simulink model "AcceleratorOld"  (R2019a)
settings: Solver=FixedStepAuto  StartTime=0.0  StopTime=20  FixedStep=step  RelTol=1e-3
model workspace (MAT data in the model file):
  a = Simulink.Signal
  a.DataType = 'double'
  a.DocUnits = 'rad/S^2'
  a.Dimensions = 1
  a.DimensionsMode = 'Fixed'
  a.Complexity = 'real'
  a.SampleTime = -1
  a.SamplingMode = 'auto'
  a.InitialValue = '0'
  d = Simulink.Signal
  d.DataType = 'double'
  d.DocUnits = 'rad'
  d.Dimensions = 1
  d.DimensionsMode = 'Fixed'
  d.Complexity = 'real'
  d.SampleTime = -1
  d.SamplingMode = 'auto'
  d.InitialValue = '0'
  j = Simulink.Signal
  j.DataType = 'double'
  j.DocUnits = 'rad/S^3'
  j.Dimensions = 1
  j.DimensionsMode = 'Fixed'
  j.Complexity = 'real'
  j.SampleTime = -1
  j.SamplingMode = 'auto'
  j.InitialValue = '1000'
  step = 0.001
  t_AASearch = Simulink.Signal
  t_AASearch.Description = 'This variable is the searching tolernece for DS.'
  t_AASearch.DataType = 'double'
  t_AASearch.DocUnits = 'm'
  t_AASearch.Dimensions = 1
  t_AASearch.DimensionsMode = 'auto'
  t_AASearch.Complexity = 'real'
  t_AASearch.SampleTime = -1
  t_AASearch.SamplingMode = 'auto'
  t_AASearch.InitialValue = '0.001'
  v = Simulink.Signal
  v.DataType = 'double'
  v.Dimensions = 1
  v.DimensionsMode = 'auto'
  v.Complexity = 'real'
  v.SampleTime = -1
  v.SamplingMode = 'auto'
  v.InitialValue = '0'
settings Model: OrderedModelArguments=off  Creator=EiLit  LastModifiedBy=EiLit
settings DataIOCC: ReturnWorkspaceOutputs=off
settings DebuggingCC: ReadBeforeWriteMsg=EnableAllAsWarning  WriteAfterWriteMsg=EnableAllAsWarning  WriteAfterReadMsg=EnableAllAsWarning  ArithmeticOperatorsInVariantConditions=warning

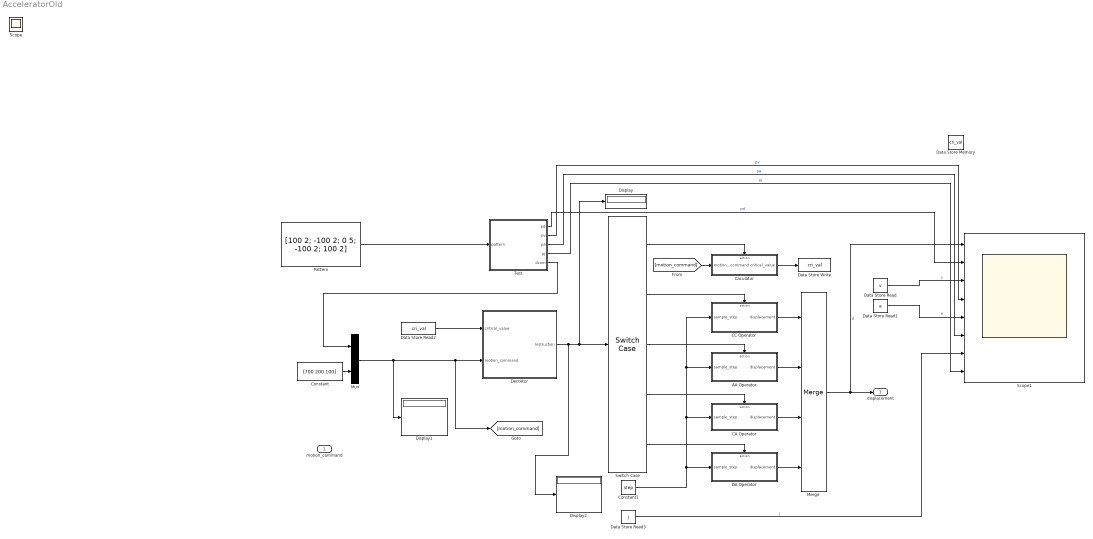
== system AcceleratorOld ==
  motion_command : Inport
  AA Operator : Subsystem  TreatAsAtomicUnit=on
  CA Operator : Subsystem  TreatAsAtomicUnit=on
  CC Operator : Subsystem  TreatAsAtomicUnit=on
  Caculator : Subsystem  TreatAsAtomicUnit=on
  Constant : Constant  Value=[700 200 100]
  Constant1 : Constant  Value=step
  DA Operator : Subsystem  TreatAsAtomicUnit=on
  Data Store Memory : DataStoreMemory  DataStoreName=cri_val  ReadBeforeWriteMsg=warning  WriteAfterWriteMsg=warning  WriteAfterReadMsg=warning  InitialValue=zeros(8,4)  ShowAdditionalParam=off
  Data Store Read : DataStoreRead  DataStoreName=v
  Data Store Read1 : DataStoreRead  DataStoreName=a
  Data Store Read2 : DataStoreRead  DataStoreName=cri_val
  Data Store Read3 : DataStoreRead  DataStoreName=j
  Data Store Write : DataStoreWrite  DataStoreName=cri_val
  Dectetor : Subsystem
  Display : Display
  Display1 : Display
  Display2 : Display
  Merge : Merge  Inputs=4  InitialOutput=[0]
  Mux : Mux  Inputs=2
  Pattern : Constant  Value=[100 2; -100 2; 0 5; -100 2; 100 2]  VectorParams1D=off
  Scope1 : Scope  NumInputPorts=8
  Switch Case : SwitchCase  CaseConditions={0,1,2,3,4}  ShowDefaultCase=off
  Test : Subsystem
  displacement : Outport
  Scope : Scope
  wires:
  Test/5(dcom) -> Mux/1
  AA Operator/1(displacement) -> Merge/2
  CC Operator/1(displacement) -> Merge/1
  Switch Case/1 -> Caculator/Action
  Data Store Read/1 -> Scope1/3  "v"
  Test/1(pd) -> Scope1/2  "pd"
  Data Store Read1/1 -> Scope1/5  "a"
  Dectetor/1(Instruction) -> Display2/1, Switch Case/1, Display/1
  Constant1/1 -> CC Operator/1(sample_step), AA Operator/1(sample_step), CA Operator/1(sample_step), DA Operator/1(sample_step)
  CA Operator/1(displacement) -> Merge/3
  DA Operator/1(displacement) -> Merge/4
  Data Store Read2/1 -> Dectetor/1(critical_value)
  Test/2(pv) -> Scope1/4  "pv"
  Switch Case/5 -> DA Operator/Action
  Merge/1 -> Scope1/1, displacement/1  "d"
  Switch Case/2 -> CC Operator/Action
  [motion_command] -> Caculator/1(motion_command)
  Caculator/1(critical_value) -> Data Store Write/1
  Constant/1 -> Mux/2
  Switch Case/3 -> AA Operator/Action
  Test/3(pa) -> Scope1/6  "pa"
  Mux/1 -> Display1/1, [motion_command], Dectetor/2(motion_command)
  Switch Case/4 -> CA Operator/Action
  Pattern/1 -> Test/1(pattern)
  Test/4(pj) -> Scope1/8  "pj"
  Data Store Read3/1 -> Scope1/7  "j"

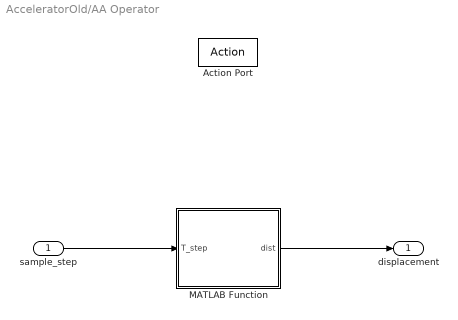
== system AcceleratorOld/AA Operator ==
  sample_step : Inport
  Action Port : ActionPort  ActionPortLabel=case [ 2 ]:
  MATLAB Function : MATLAB Function  TreatAsAtomicUnit=on
  displacement : Outport  PortDimensions=1
  wires:
  sample_step/1 -> MATLAB Function/1(T_step)
  MATLAB Function/1(dist) -> displacement/1

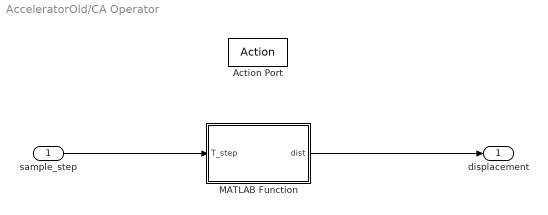
== system AcceleratorOld/CA Operator ==
  sample_step : Inport
  Action Port : ActionPort  ActionPortLabel=case [ 3 ]:
  MATLAB Function : MATLAB Function  TreatAsAtomicUnit=on
  displacement : Outport
  wires:
  sample_step/1 -> MATLAB Function/1(T_step)
  MATLAB Function/1(dist) -> displacement/1

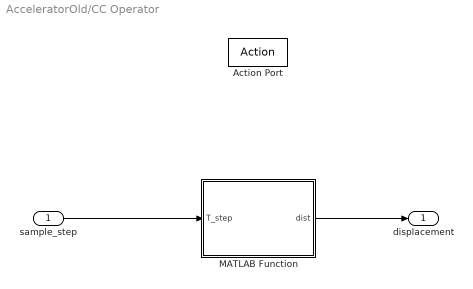
== system AcceleratorOld/CC Operator ==
  sample_step : Inport
  Action Port : ActionPort  ActionPortLabel=case [ 1 ]:
  MATLAB Function : MATLAB Function  TreatAsAtomicUnit=on
  displacement : Outport
  wires:
  MATLAB Function/1(dist) -> displacement/1
  sample_step/1 -> MATLAB Function/1(T_step)

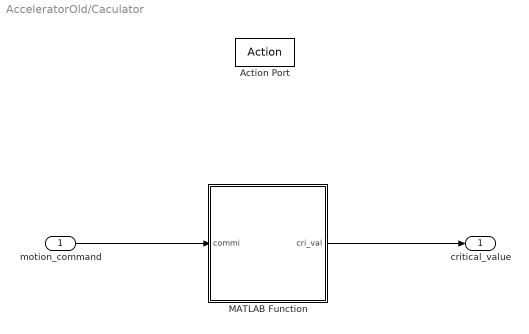
== system AcceleratorOld/Caculator ==
  motion_command : Inport
  Action Port : ActionPort  ActionPortLabel=case [ 0 ]:
  MATLAB Function : MATLAB Function  TreatAsAtomicUnit=on
  critical_value : Outport
  wires:
  motion_command/1 -> MATLAB Function/1(commi)
  MATLAB Function/1(cri_val) -> critical_value/1

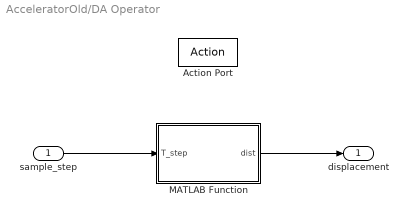
== system AcceleratorOld/DA Operator ==
  sample_step : Inport
  Action Port : ActionPort  ActionPortLabel=case [ 4 ]:
  MATLAB Function : MATLAB Function  TreatAsAtomicUnit=on
  displacement : Outport
  wires:
  sample_step/1 -> MATLAB Function/1(T_step)
  MATLAB Function/1(dist) -> displacement/1

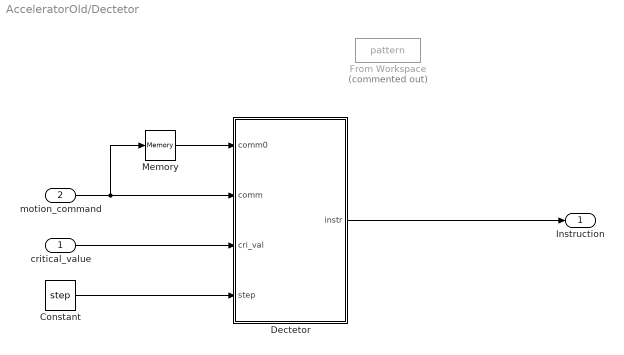
== system AcceleratorOld/Dectetor ==
  critical_value : Inport
  motion_command : Inport  Port=2
  Constant : Constant  Value=step
  Dectetor : MATLAB Function  TreatAsAtomicUnit=on
  From Workspace : FromWorkspace  Commented=on  VariableName=pattern  SampleTime=0
  Memory : Memory  InitialCondition=[0 0 0 0]
  Instruction : Outport
  wires:
  motion_command/1 -> Memory/1, Dectetor/2(comm)
  Dectetor/1(instr) -> Instruction/1
  critical_value/1 -> Dectetor/3(cri_val)
  Memory/1 -> Dectetor/1(comm0)
  Constant/1 -> Dectetor/4(step)

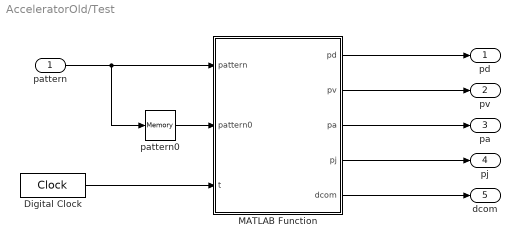
== system AcceleratorOld/Test ==
  pattern : Inport
  Digital Clock : DigitalClock  SampleTime=0.001
  MATLAB Function : MATLAB Function  TreatAsAtomicUnit=on
  pattern0 : Memory
  pd : Outport
  pv : Outport  Port=2
  pa : Outport  Port=3
  pj : Outport  Port=4
  dcom : Outport  Port=5
  wires:
  pattern/1 -> MATLAB Function/1(pattern), pattern0/1
  MATLAB Function/1(pd) -> pd/1
  pattern0/1 -> MATLAB Function/2(pattern0)
  Digital Clock/1 -> MATLAB Function/3(t)
  MATLAB Function/4(pj) -> pj/1
  MATLAB Function/3(pa) -> pa/1
  MATLAB Function/2(pv) -> pv/1
  MATLAB Function/5(dcom) -> dcom/1

== matlab function AcceleratorOld/Dectetor/Dectetor ==
  data: comm0 input; comm input; instr output; cri_val input; d data_store_memory; v data_store_memory; a data_store_memory; step input; j data_store_memory
function instr = fcn(comm0, comm, cri_val, step)
%% Initialization
global d v a j
persistent phasei

instr = 0;

if isempty(phasei)
    phasei = 0;
end

% i stands for ith step:
% step 0: pre-Acc step;
% step 1: 1st Acc step;
% step 2: 1st CA step;
% step 3: 1st Dec step;
% ...

% Judge the direction
dir = comm(1)/abs(comm(1));
comm(2:4) = dir * comm(2:4);
commabs = abs(comm);            % Absolute command value used to calculate the neighbor.

%% Determine the instruction
if ~(comm == comm0)                % If need to re-calculate the critical value.
    instr = 0;
    j = 0;
    phasei = 0;
else
    temp1 = cri_val(2,3) - commabs(4) * step;      % The neighbor of the critical value used to take care of the direction of acceleration of the 1st step
    temp2 = cri_val(2,3) + commabs(4) * step;
    switch phasei
        case 0
            if cri_val(1,3)==0    % If there is pre-Acc step exist (or intially 0)
                if a*(a+comm(4)*step) >= 0    %If the pre-Acc step finished
                    [d, v, a, j, phasei, instr] = instrGen(step, dir, phasei, instr, cri_val, comm, commabs, temp1, temp2);
                else                        %If the pre-Acc step not finished
                    instr = 2;
                    j = -comm(4);
                end
            else                            %If the pre-Acc step does not exist
                [d, v, a, j, phasei, instr] = instrGen(step, dir, phasei, instr, cri_val, comm, commabs, temp1, temp2);
            end
        case 1
            if temp1<=a && a<=temp2                  % If a is in the neighbor, then step 1 is finished.
                [d, v, a, j, phasei, instr] = instrGen(step, dir, phasei, instr, cri_val, comm, commabs, temp1, temp2);
            else
                instr = 2;
                if a > cri_val(2,3)
                    j = -commabs(4);
                else
                    j = commabs(4);
                end
            end
        case 2
            temp = v + 0.5*comm(4)*step^2 + cri_val(3,3)*step;
            if dir * temp >= dir * cri_val(3,2)     % If velocity reaches the critical value
                [d, v, a, j, phasei, instr] = instrGen(step, dir, phasei, instr, cri_val, comm, commabs, temp1, temp2);
            else                                    % If velocity does not reach the critical value
                j = 0;
                instr = 3;
            end
        case 3
            temp = a - comm(4) * step;
            if dir * temp <= 0            % If acceleration is reduced to 0;
                [d, v, a, j, phasei, instr] = instrGen(step, dir, phasei, instr, cri_val, comm, commabs, temp1, temp2);
            else                                    % If acceleration is not reduced to 0;
                j = comm(4);
                instr = 4;
            end
        case 4
            temp = d + cri_val(5,2)*step;
            if dir * temp >= dir * cri_val(5,1)
                [d, v, a, j, phasei, instr] = instrGen(step, dir, phasei, instr, cri_val, comm, commabs, temp1, temp2);
            else
                j = 0;
                instr = 1;
            end
        case 5
            temp = a - comm(4) * step;
            if dir * temp <= dir * cri_val(6,3)
                [d, v, a, j, phasei, instr] = instrGen(step, dir, phasei, instr, cri_val, comm, commabs, temp1, temp2);
            else
                j = -comm(4);
                instr = 2;
            end
        case 6
            temp = v - 0.5*comm(4)*step^2 + cri_val(7,3)*step;
            if dir * temp <= cri_val(7,2)
                [d, v, a, j, phasei, instr] = instrGen(step, dir, phasei, instr, cri_val, comm, commabs, temp1, temp2);
            else
                j = 0;
                instr = 3;
            end
        case 7
            temp = a + comm(4) * step;
            if dir * temp >= 0
                [d, v, a, j, phasei, instr] = instrGen(step, dir, phasei, instr, cri_val, comm, commabs, temp1, temp2);
            else
                j = -comm(4);
                instr = 4;
            end
        otherwise
            instr = 1;
            j = 0;
    end
end
  
end

== matlab function AcceleratorOld/CC Operator/MATLAB Function ==
  data: T_step input; dist output; v data_store_memory; d data_store_memory; a data_store_memory
function dist = fcn(T_step)
global d v a
a = 0;
d = d + v*T_step;
dist = d;

== matlab function AcceleratorOld/AA Operator/MATLAB Function ==
  data: T_step input; dist output; d data_store_memory; v data_store_memory; a data_store_memory; j data_store_memory
function dist = fcn(T_step)
global d v a j
a = a + j*T_step;
v = v + a*T_step + 1/2*j*T_step^2;
d = d + v*T_step + 1/2*a*T_step^2 + 1/6*j*T_step^3;
dist = d;

== matlab function AcceleratorOld/CA Operator/MATLAB Function ==
  data: T_step input; dist output; d data_store_memory; v data_store_memory; a data_store_memory
function dist = fcn(T_step)
global d v a
v = v + a*T_step;
d = d + v*T_step + 1/2*a*T_step^2;
dist = d;

== matlab function AcceleratorOld/DA Operator/MATLAB Function ==
  data: T_step input; dist output; d data_store_memory; v data_store_memory; a data_store_memory; j data_store_memory
function dist = fcn(T_step)
global d v a j
a = a - j*T_step;
v = v + a*T_step - 1/2*j*T_step^2;
d = d + v*T_step + 1/2*a*T_step^2 - 1/6*j*T_step^3;
dist = d;

== matlab function AcceleratorOld/Caculator/MATLAB Function ==
  data: commi input; d data_store_memory; v data_store_memory; a data_store_memory; cri_val output; t_AASearch data_store_memory
function cri_val = fcn(commi)
%% Preprocess
global d v a t_AASearch
% Reset the displacement
d = 0;

% Deal with the direction.
comm = commi;
if commi(1) < 0
    comm = -abs(comm);
end

%% Deal with the pre-acceleration process
% This pre phase should be dealed with at the first step, as it is fixed.
pre_cr = Pre_Acc(comm, d, v, a);

%% Velocity Shortage Determination
% The difference judgement is used, as the correction need the jerk.
% Compute the modified command.
comm_velmod = VelS_ComCal(comm,pre_cr);

%% 1st Standard Process Calculation
% This is to calculate the critical values for the standard
% process. Based on these values, further determination can be made.
[d_cr, v_cr, a_cr, t_cr] = Std_PRO_cr(comm_velmod, pre_cr);    
    
%% Displacement Shortage Determination
DS_flag = DisS_Judge(d_cr,comm);

if DS_flag
    d_cr(5:8) = d_cr(5:8) - d_cr(5) + d_cr(4);
    [Ind,ds_cr,vs_cr,as_cr,ts_cr] = DisS_CJ(d_cr,comm_velmod,pre_cr);
    switch Ind
        case 1          %The DS can't be made up
            d_cr = ds_cr;
            v_cr = vs_cr;
            a_cr = as_cr;
            t_cr = ts_cr;
        case 2          %The DS can be made up by modifing the CA step
            [d_cr, v_cr, a_cr, t_cr] = DisS_CAModiCal(d_cr,v_cr,t_cr,comm_velmod,pre_cr);
        case 3          %The DS can be made up by changing the acceleration
            dis_comm = comm_velmod;
            if length(comm_velmod) < 5          % If is feedrate shortage
                dis_comm(2) = dis_comm(2) - min(v_cr(3)-v_cr(2), v_cr(7)-v_cr(6));
            end
            [d_cr, v_cr, a_cr, t_cr] = DisS_AAModiCal(dis_comm, pre_cr, t_AASearch);
    end
end

%% Postprocess
cri_val = [d_cr', v_cr', a_cr', t_cr'];
end

== matlab function AcceleratorOld/Test/MATLAB Function ==
  data: pattern input; pd output; pattern0 input; pv output; pa output; pj output; d data_store_memory; v data_store_memory; a data_store_memory; t input; dcom output
function [pd, pv, pa, pj, dcom] = fcn(pattern, pattern0, t)
global d v a
persistent t0 d0 v0 a0 dcom_temp

if isempty(t0)
        t0 = 0;
        d0 = 0;
        v0 = 0;
        a0 = 0;
        dcom_temp = 0;
end

if ~(pattern == pattern0)
    d0 = d;
    v0 = v;
    a0 = a;
    t0 = t;
    [plotData, ~] = ProfileGenerator(pattern,d0,v0,a0);
    dcom_temp = plotData(1,end);
end

[pd, pv, pa, pj] = ProfileGeneratorT(pattern,d0,v0,a0,t-t0);
dcom = dcom_temp;
